simulink model "vlsi_single_pll"  (R2020a)
settings: Solver=ode45  StartTime=0.0  StopTime=10e-5  RelTol=1e-3  EnableMultiTasking=on
values from neighbouring files (symbols this model uses):
  f0_dco = f0_dco0+gain_dco0*rand()    [pll_Nbit_vlsi_init.m]
  freq_ref = 2.227965e8    (= 222796500)    [pll_Nbit_vlsi_init.m]
  gain_dco = gain_dco0*(1+0.00*(rand-0.5))    [pll_Nbit_vlsi_init.m]
  integrator_init_state = Kint_den*(integrator_init_state_min+ 0.1*(integrator_init_state_max-integrator_init_state_min))    (= 419020.8)    [pll_Nbit_vlsi_init.m]
  phi0 = rand*2*pi    [pll_Nbit_vlsi_init.m]
libraries: library_adpll x2
settings Model: Creator=galayko  LastModifiedBy=galayko
settings DataIOCC: LimitDataPoints=on  SaveFormat=Array  SignalLoggingSaveFormat=ModelDataLogs  ReturnWorkspaceOutputs=off
settings OptimizationCC: ConditionallyExecuteInputs=off  ExpressionDepthLimit=2147483647  LifeSpan=inf  SimCompilerOptimization=on  AccelVerboseBuild=on
settings DebuggingCC: UnderspecifiedInitializationDetection=Classic  MergeDetectMultiDrivingBlocksExec=none  MaxConsecutiveZCsMsg=warning  SolverPrmCheckMsg=warning  MultiTaskRateTransMsg=warning  FcnCallInpInsideContextMsg=warning  ModelReferenceIOMsg=warning  ModelReferenceVersionMismatchMessage=warning  ModelReferenceIOMismatchMessage=warning  ModelReferenceExtraNoncontSigs=warning  StateNameClashWarn=warning  SFUnexpectedBacktrackingDiag=warning  SFNoUnconditionalDefaultTransitionDiag=warning  ArithmeticOperatorsInVariantConditions=warning
settings HardwareCC: ProdBitPerPointer=32  ProdBitPerSizeT=32  ProdBitPerPtrDiffT=32  ProdLargestAtomicFloat=None  ProdIntDivRoundTo=Undefined  ProdEndianess=Unspecified  ProdWordSize=32  ProdHWDeviceType=32-bit Generic
settings ModelReferenceCC: PropagateSignalLabelsOutOfModel=off
settings SFSimCC: SimUseLocalCustomCode=off  SimParseCustomCode=off  CustomCodeUndefinedFunction=UseInterfaceOnly
settings RTWCC: RTWUseLocalCustomCode=off
settings CodeAppCC: StateflowObjectComments=on
settings GRTTargetCC: TargetLangStandard=C89/C90 (ANSI)  CombineOutputUpdateFcns=off  GRTInterface=on
settings ConfigComp: CovMetricSettings=dw  CovHtmlReporting=on  CovSaveCumulativeToWorkspaceVar=on  CovSaveSingleToWorkspaceVar=on  CovExternalEMLEnable=off  CovSFcnEnable=off

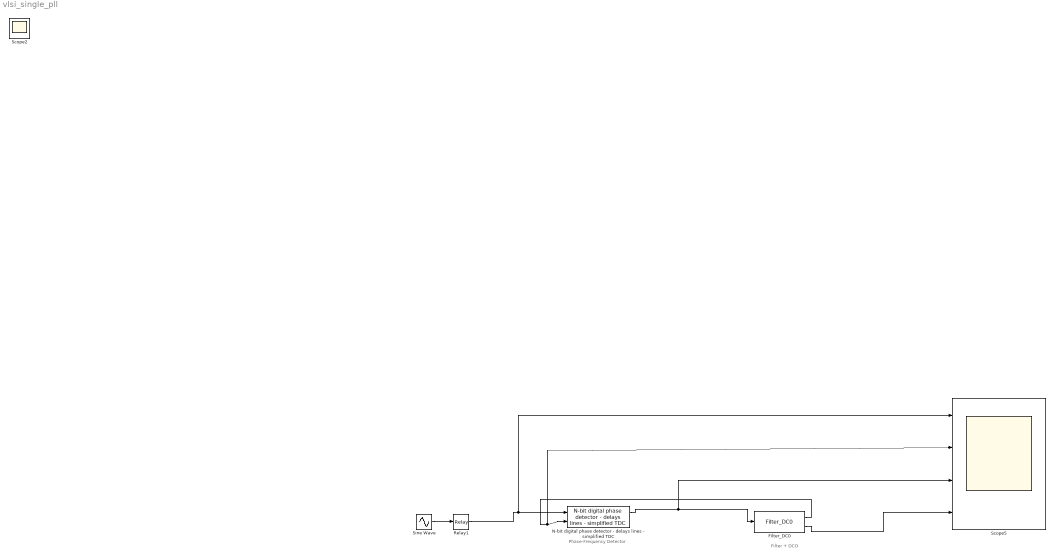
== system vlsi_single_pll ==
  note: Filter + DCO
  note: Phase-Frequency Detector
  Filter_DC0 : library_adpll/Filter_DC0  Kprop_num=Kprop_num  Kprop_den=Kprop_den  Kint_num=Kint_num  Kint_den=Kint_den  f0_dco=f0_dco(1)  gain_dco=gain_dco(1)  phi0=phi0(1)  integrator_init_state=integrator_init_state(1)  Nprop_out=Nprop_out  Nprop_in=Nprop_in
      link override Triggered Subsystem3/Out1: InitialOutput=0
  N-bit digital phase detector - delays lines - simplified TDC : library_adpll/N-bit digital phase detector - delays lines - simplified TDC  T0=32e-12  D=0
  Relay1 : Relay  OnSwitchValue=0  OffSwitchValue=0  OffOutputValue=-1
  Scope5 : Scope  NumInputPorts=4
  Sine Wave : Sin  Frequency=2*pi*freq_ref  SampleTime=0
  Scope2 : Scope
  wires:
  N-bit digital phase detector - delays lines - simplified TDC/1 -> Filter_DC0/1, Scope5/3
  Relay1/1 -> N-bit digital phase detector - delays lines - simplified TDC/1, Scope5/1
  Sine Wave/1 -> Relay1/1
  Filter_DC0/1 -> N-bit digital phase detector - delays lines - simplified TDC/2, Scope5/2
  Filter_DC0/2 -> Scope5/4
